simulink model "PID_example"  (R2018b)
settings: Solver=ode4  StartTime=0.0  StopTime=10.0  FixedStep=0.0001  RelTol=1e-3
settings Model: Creator=carlos  LastModifiedBy=carlos

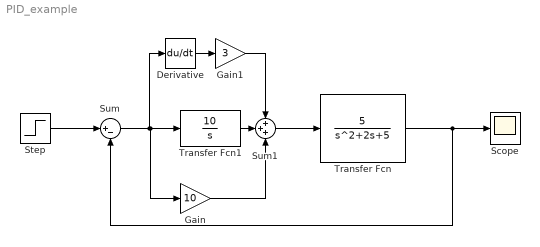
== system PID_example ==
  Derivative : Derivative
  Gain : Gain  Gain=10
  Gain1 : Gain  Gain=3
  Scope : Scope
  Step : Step  Time=0  SampleTime=0
  Sum : Sum  Inputs=|+-
  Sum1 : Sum  Inputs=+++
  Transfer Fcn : TransferFcn  Numerator=[5]  Denominator=[1 2 5]
  Transfer Fcn1 : TransferFcn  Numerator=10  Denominator=[1 0]
  wires:
  Transfer Fcn/1 -> Sum/2, Scope/1
  Sum/1 -> Transfer Fcn1/1, Gain/1, Derivative/1
  Step/1 -> Sum/1
  Derivative/1 -> Gain1/1
  Gain1/1 -> Sum1/1
  Sum1/1 -> Transfer Fcn/1
  Gain/1 -> Sum1/3
  Transfer Fcn1/1 -> Sum1/2
